simulink model "Bidirectional"  (R2024b)
settings: Solver=ode1  StartTime=0.0  StopTime=4  FixedStep=1e-6  RelTol=1e-3
undefined symbols (not defined in the file): Acid, Lead
libraries: spsSeriesRLCBranchLib x4, spsVoltageMeasurementLib x3, simulink x2, spsCurrentMeasurementLib x2, spsIGBTDiodeLib x2, spsBatteryLib x1, spsBreakerLib x1, sps_lib x1
settings Model: Creator=Ashwin Soni  LastModifiedBy=Ashwin Soni

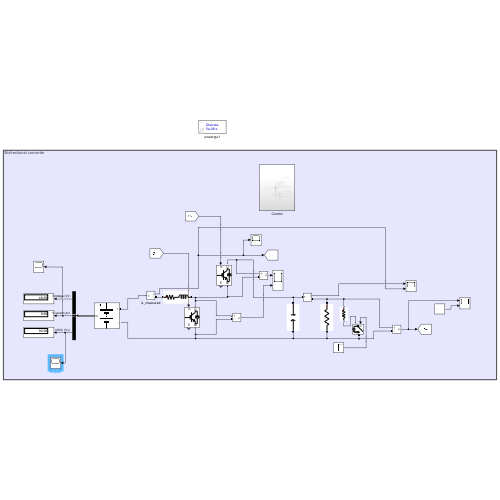
[thumbnail: Simulink's stored preview of the top-level diagram]
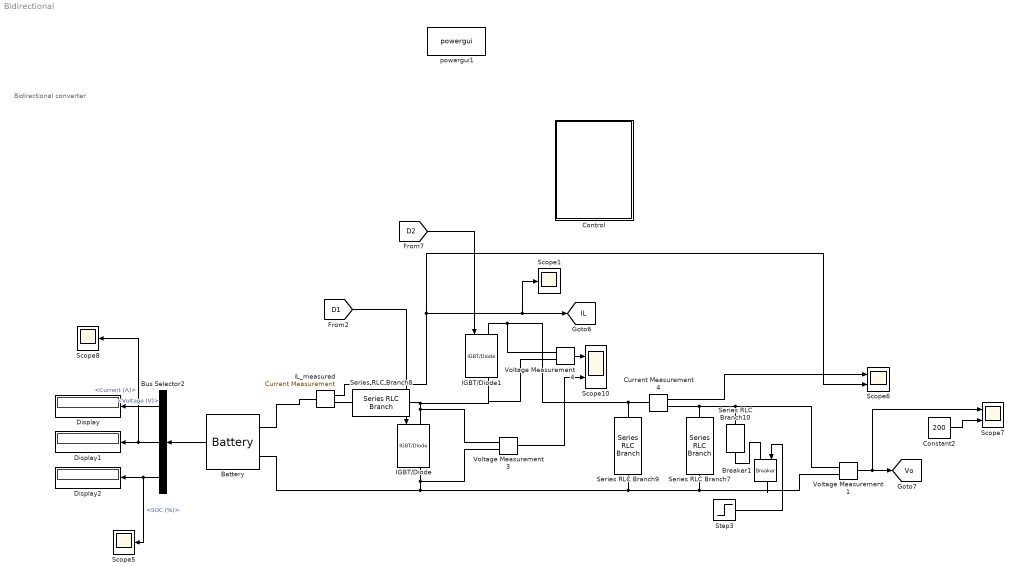
== system Bidirectional ==
  note: Bidirectional converter
  Battery : spsBatteryLib/Battery  BatType=Lead-Acid  NomV=48  NomQ=26  SOC=90  Batt_Tr=30  PresetModel=on  MaxQ=27.0833  MinV=36  FullV=52.2632  Dis_rate=5.2  R=0.018462  Normal_OP=8.0672  expZone="[48.8684    0.0866667]"
  Breaker1 : spsBreakerLib/Breaker  InitialState=0  SwitchingTimes="[1/60  5/60]"  External=on  BreakerResistance=0.01  SnubberResistance=1e6  SnubberCapacitance=inf  Measurements=None  MoreParameters=on  NoBreakLoop=off
  Bus Selector2 : BusSelector  OutputSignals=Voltage (V),Current (A),SOC (%)
  Constant2 : Constant  Value=200
  Control : Subsystem
  Current Measurement4 : spsCurrentMeasurementLib/Current Measurement  PhasorSimulation=off  OutputType=Complex  PSBequivalent=0
  Display : Display
  Display1 : Display
  Display2 : Display
  IGBT/Diode : spsIGBTDiodeLib/IGBT//Diode  Ron=1e-3  Rs=5  Cs=15e-9  Measurements=on
  IGBT/Diode1 : spsIGBTDiodeLib/IGBT//Diode  Ron=1e-3  Rs=5  Cs=15e-9  Measurements=on
  Scope1 : Scope
  Scope10 : Scope  NumInputPorts=2
  Scope5 : Scope
  Scope6 : Scope  NumInputPorts=2
  Scope7 : Scope  NumInputPorts=2
  Scope8 : Scope
  Series RLC Branch10 : spsSeriesRLCBranchLib/Series RLC Branch  LConnTagsString=__new0  RConnTagsString=__new0  BranchType=R  Resistance=200  Inductance=10e-3  SetiL0=off  InitialCurrent=0  Capacitance=1e-6  Setx0=off  InitialVoltage=0  Measurements=None
  Series RLC Branch7 : spsSeriesRLCBranchLib/Series RLC Branch  LConnTagsString=__new0  RConnTagsString=__new0  BranchType=R  Resistance=160  Inductance=10e-3  SetiL0=off  InitialCurrent=0  Capacitance=1e-6  Setx0=off  InitialVoltage=0  Measurements=None
  Series RLC Branch8 : spsSeriesRLCBranchLib/Series RLC Branch  LConnTagsString=__new0  RConnTagsString=__new0  BranchType=RL  Resistance=0.2  Inductance=6.67e-3  SetiL0=off  InitialCurrent=0  Capacitance=1e-6  Setx0=off  InitialVoltage=0  Measurements=None
  Series RLC Branch9 : spsSeriesRLCBranchLib/Series RLC Branch  LConnTagsString=__new0  RConnTagsString=__new0  BranchType=C  Resistance=1  Inductance=1e-3  SetiL0=off  InitialCurrent=0  Capacitance=440e-6  Setx0=off  InitialVoltage=0  Measurements=None
  Step3 : Step  Time=2  SampleTime=0
  Voltage Measurement1 : spsVoltageMeasurementLib/Voltage Measurement  PhasorSimulation=off  OutputType=Complex  PSBequivalent=0
  Voltage Measurement3 : spsVoltageMeasurementLib/Voltage Measurement  PhasorSimulation=off  OutputType=Complex  PSBequivalent=0
  Voltage Measurement4 : spsVoltageMeasurementLib/Voltage Measurement  PhasorSimulation=off  OutputType=Complex  PSBequivalent=0
  iL_measured : spsCurrentMeasurementLib/Current Measurement  PhasorSimulation=off  OutputType=Complex  PSBequivalent=0
  powergui1 : sps_lib/powergui  Priority=1  SimulationMode=Discrete  SampleTime=5e-6  frequency=60  Iterations=50  frequencyindice=0  Pbase=100e6  ErrMax=1e-4  UnitsV=kV  UnitsW=MW  buscounter=0  FunctionMessages=off  echomessages=off  EnableUseOfTLC=off  CurrentSourceSwitches=off  DisableSnubberDevices=off  DisableRonSwitches=off  DisableVfSwitches=off  DisplayEquations=off  AutomaticDiscreteSolvers=off  SolverType=Tustin/Backward Euler (TBE)  Interpol=off  ExternalGateDelay=off  methode=off  Ts=100  x0status=blocks  SPID=on  SwTol=0  HookPort=off  NonlinearTolerance=1e-4  nMaxIteration=100  ContinueOnMaxIteration=off  RestoreLinks=warning  ResistiveCurrentMeasurement=off  Frange=[0:2:500]  Ylog=off  Xlog=on  ShowGrid=off  save=off  variable=ZData  structure=0  ZoomFFT=off  StartTime=0.0  cycles=1  DisplayStyle=1  fundamental=60  FreqAxis=off  MaxFrequency=1000  frequencyindicesteady=1  RmsSteady=1  display=off
  tag scope: IL=global, Vo=global
  wires:
  Bus Selector2/3 -> Scope5/1, Display2/1  "<SOC (%)>"
  Bus Selector2/1 -> Display/1  "<Voltage (V)>"
  Voltage Measurement1/1 -> Scope7/1, [Vo]
  Step3/1 -> Breaker1/1
  Battery/1 -> Bus Selector2/1
  Constant2/1 -> Scope7/2
  Voltage Measurement4/1 -> Scope10/1
  [D2] -> IGBT/Diode1/1
  iL_measured/1 -> Scope1/1, [IL], Scope6/2
  Voltage Measurement3/1 -> Scope10/2
  [D1] -> IGBT/Diode/1
  Current Measurement4/1 -> Scope6/1
  Bus Selector2/2 -> Scope8/1, Display1/1  "<Current (A)>"
  connections:
  IGBT/Diode/LConn1 -- Voltage Measurement3/LConn1 -- Voltage Measurement4/LConn2 -- IGBT/Diode1/RConn1 -- Series RLC Branch8/RConn1
  Voltage Measurement4/LConn1 -- Series RLC Branch9/LConn1 -- Current Measurement4/LConn1 -- IGBT/Diode1/LConn1
  IGBT/Diode/RConn1 -- Voltage Measurement1/LConn2 -- Breaker1/RConn1 -- Series RLC Branch7/RConn1 -- Series RLC Branch9/RConn1 -- Battery/LConn2 -- Voltage Measurement3/LConn2
  Series RLC Branch10/LConn1 -- Series RLC Branch7/LConn1 -- Current Measurement4/RConn1 -- Voltage Measurement1/LConn1
  Breaker1/LConn1 -- Series RLC Branch10/RConn1
  iL_measured/RConn1 -- Series RLC Branch8/LConn1
  Battery/LConn1 -- iL_measured/LConn1

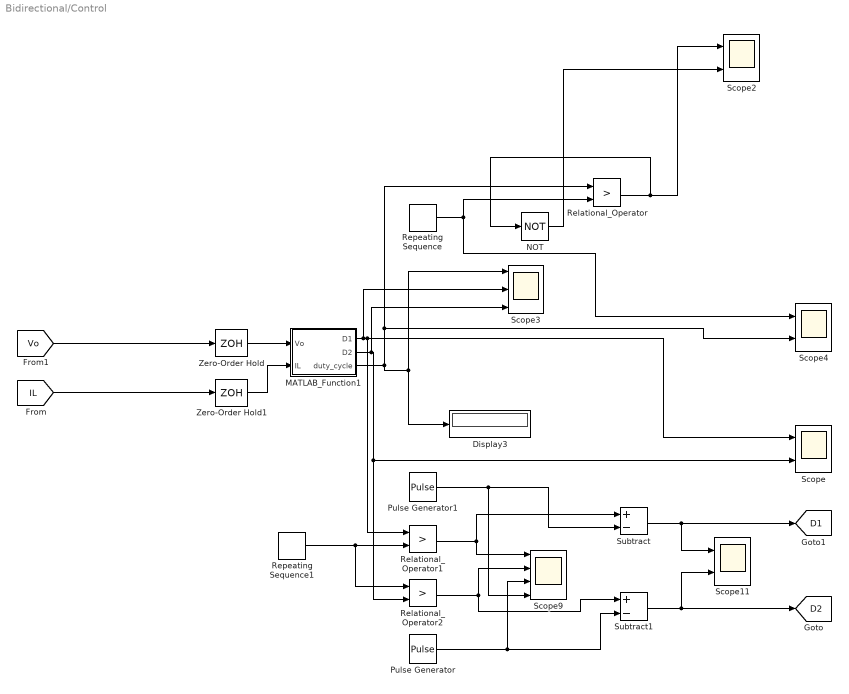
== system Bidirectional/Control ==
  Display3 : Display
  MATLAB_Function1 : MATLAB Function  TreatAsAtomicUnit=on
  NOT : Logic  Operator=NOT  IconShape=distinctive  AllPortsSameDT=off  OutDataTypeStr=boolean
  Pulse Generator : DiscretePulseGenerator  PulseType=Time based  Period=1e-4  PulseWidth=5  PhaseDelay=-5e-6
  Pulse Generator1 : DiscretePulseGenerator  PulseType=Time based  Period=1e-4  PulseWidth=5
  Relational_Operator : RelationalOperator  Operator=>  OutDataTypeStr=boolean  RndMeth=Simplest  InputSameDT=off
  Relational_Operator1 : RelationalOperator  Operator=>  OutDataTypeStr=boolean  RndMeth=Simplest  InputSameDT=off
  Relational_Operator2 : RelationalOperator  Operator=>  OutDataTypeStr=boolean  RndMeth=Simplest  InputSameDT=off
  Repeating Sequence : simulink/Sources/Repeating Sequence  rep_seq_t=[0 0.5 1]*(1/(10e3))  rep_seq_y=[0 1 0]
  Repeating Sequence1 : simulink/Sources/Repeating Sequence  rep_seq_t=[0 1]*(1/(10e3))  rep_seq_y=[0 1]
  Scope{,2,4,11} (4 alike) : Scope  NumInputPorts=2
  Scope3 : Scope  NumInputPorts=3
  Scope9 : Scope  NumInputPorts=4
  Subtract : Sum  Inputs=+-
  Subtract1 : Sum  Inputs=+-
  Zero-Order Hold : ZeroOrderHold  SampleTime=1e-4
  Zero-Order Hold1 : ZeroOrderHold  SampleTime=1e-4
  tag scope: D1=global, D2=global
  wires:
  Repeating Sequence/1 -> Scope4/1, Relational_Operator/2
  Subtract1/1 -> [D2], Scope11/2
  Zero-Order Hold/1 -> MATLAB_Function1/1(Vo)
  Subtract/1 -> [D1], Scope11/1
  MATLAB_Function1/3(duty_cycle) -> Scope3/1, Display3/1, Relational_Operator/1, Scope4/2
  Relational_Operator1/1 -> Subtract/1, Scope9/1
  Pulse Generator1/1 -> Scope9/4, Subtract/2
  Repeating Sequence1/1 -> Relational_Operator2/1, Relational_Operator1/2
  Relational_Operator2/1 -> Subtract1/1, Scope9/2
  Zero-Order Hold1/1 -> MATLAB_Function1/2(IL)
  [IL] -> Zero-Order Hold1/1
  MATLAB_Function1/1(D1) -> Scope3/2, Relational_Operator1/1, Scope/1
  MATLAB_Function1/2(D2) -> Scope3/3, Relational_Operator2/2, Scope/2
  NOT/1 -> Scope2/2
  Relational_Operator/1 -> NOT/1, Scope2/1
  [Vo] -> Zero-Order Hold/1
  Pulse Generator/1 -> Scope9/3, Subtract1/2

== matlab function Bidirectional/Control/MATLAB_Function1 ==
  data: D1 output; D2 output; Vo input; IL input; duty_cycle output
function [D1,D2,duty_cycle]  = control(Vo, IL)
    % Constants
    V_ref = 200;                % Reference voltage (400V)
    Kp_v = 0.1;                 % Proportional gain for voltage PI controller
    Ki_v = 8;               % Integral gain for voltage PI controller
    Kp_i = 0.02;                 % Proportional gain for current PI controller
    Ki_i = 5;              % Integral gain for current PI controller
    dead_duty = 5e-6/1e-4;           % Dead time in seconds (adjust as needed)

    %% Corrected this Ts recently as per 10kHz sampling, need to tune the pi values again;
    Ts = 1e-4;                  % Sampling time in seconds

    % Persistent variables for integrators
   % Persistent variables for integrators
    persistent error_v_int error_i_int count I_ref_old first_time_entry windup;
    if isempty(error_v_int)
        error_v_int = 0;
        error_i_int = 0;
        count = 0;
        I_ref_old = 0;
        first_time_entry = 0;
        windup = 0;
    end
    
    if(first_time_entry == 0)
        first_time_entry = 1;
        error_v = V_ref - Vo;       % Voltage error
        error_v_int = error_v_int + (error_v * Ts * 1);  % Integrate the voltage error
        I_ref = (Kp_v * error_v) + (Ki_v * error_v_int);  % Output: Current reference
        I_ref_old = I_ref;
    end

    % Voltage Control Loop (Outer Loop)
    if(count == 50)
        error_v = V_ref - Vo;       % Voltage error
        error_v_int = error_v_int + (error_v * Ts * count);  % Integrate the voltage error
        I_ref = (Kp_v * error_v) + (Ki_v * error_v_int);  % Output: Current reference
        I_ref_old = I_ref;
        count = 0;
    else 
        I_ref = I_ref_old;
    end
    
    % Temporary for innerloop tuning
    %I_ref = 7;

    % Current Control Loop (Inner Loop)
    error_i = I_ref - IL + windup;       % Current error
    error_i_int = error_i_int + (error_i * Ts);  % Integrate the current error
    duty_cycle = (Kp_i * error_i) + (Ki_i * error_i_int);  % Output: Duty cycle
    
    % Clamp duty cycle to [0, 1]
    duty = max(0.05, min(0.95, duty_cycle));

    windup = duty - duty_cycle;

    % % Dead Time Logic DONT WRITE THIS IN C2000 CODE AS IT IS TO BE
    % HANDELED BY C2000 HARDWARE AND NOT BY OUR FUNCTION 
    
    D1 = duty - (dead_duty/2);
    D2 = duty + (dead_duty/2);

    count = count + 1;
    
end
